simulink library "stateMachine_lib"  (R2022b)
settings: Solver=VariableStepAuto  StartTime=0.0  StopTime=10.0  RelTol=1e-3
settings Model: Creator=serga  LastModifiedBy=serga

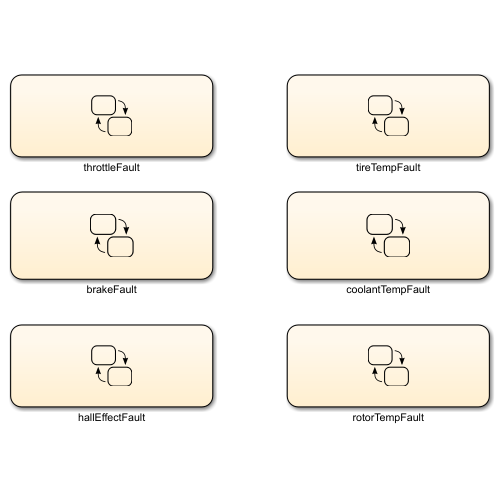
[thumbnail: Simulink's stored preview of the top-level diagram]
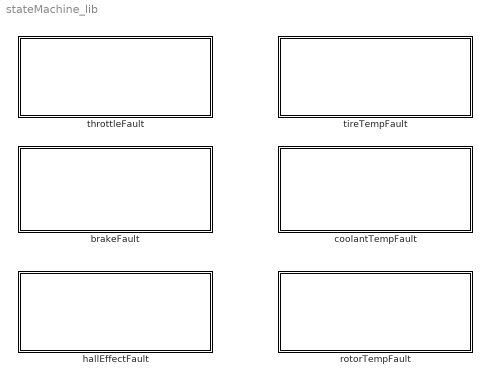
== system stateMachine_lib ==
  brakeFault : Stateflow chart  TreatAsAtomicUnit=on
  coolantTempFault : Stateflow chart  TreatAsAtomicUnit=on
  hallEffectFault : Stateflow chart  TreatAsAtomicUnit=on
  rotorTempFault : Stateflow chart  TreatAsAtomicUnit=on
  throttleFault : Stateflow chart  TreatAsAtomicUnit=on
  tireTempFault : Stateflow chart  TreatAsAtomicUnit=on

== stateflow chart stateMachine_lib/coolantTempFault ==

== stateflow chart stateMachine_lib/rotorTempFault ==

== stateflow chart stateMachine_lib/brakeFault ==

== stateflow chart stateMachine_lib/hallEffectFault ==

== stateflow chart stateMachine_lib/throttleFault ==

== stateflow chart stateMachine_lib/tireTempFault ==
